simulink model "systeme_sol_2017a_PID_v1"  (R2017a)
settings: Solver=VariableStepAuto  StartTime=0.0  StopTime=50000  RelTol=1e-3
libraries: simulink x2
settings Model: Creator=julien  LastModifiedBy=admin
settings DataIOCC: ReturnWorkspaceOutputs=on
settings SFSimCC: SimUseLocalCustomCode=on
settings RTWCC: RTWUseLocalCustomCode=on

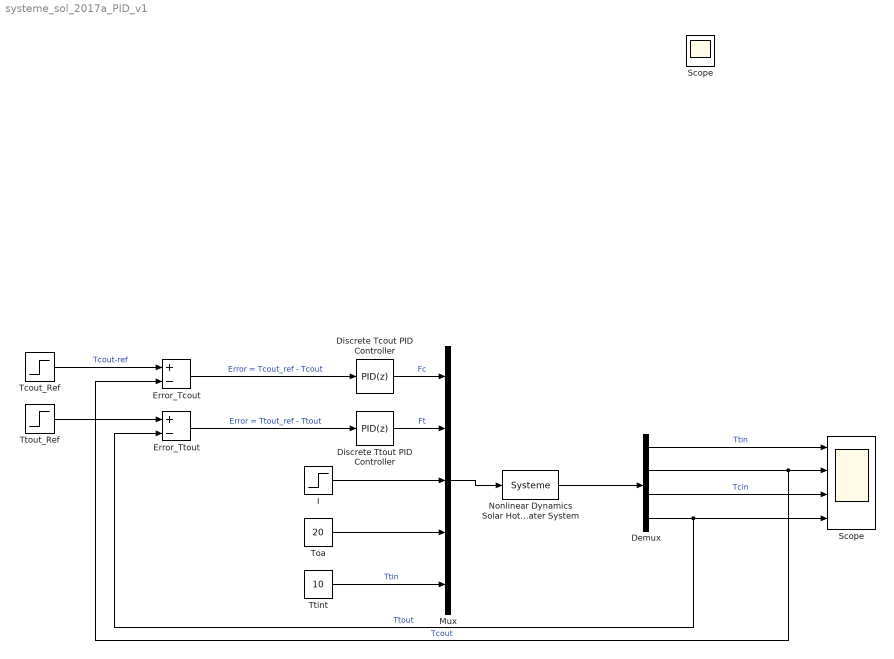
== system systeme_sol_2017a_PID_v1 ==
  Demux : Demux
  Discrete Tcout PID Controller : simulink/Continuous/PID Controller  Controller=PID  TimeDomain=Discrete-time  SampleTime=-1  IntegratorMethod=Forward Euler  FilterMethod=Forward Euler  Form=Ideal  UseFilter=on  ControllerParametersSource=internal  P=-0.0001  I=0  D=0  N=100  InitialConditionSource=internal  InitialConditionForIntegrator=0  InitialConditionForFilter=0  ExternalReset=none  LimitOutput=on  UpperSaturationLimit=2.5e-5  LowerSaturationLimit=0  LinearizeAsGain=off  AntiWindupMode=none  Kb=1  TrackingMode=off  Kt=1  PParamMin=[]  PParamMax=[]  IParamMin=[]  IParamMax=[]  DParamMin=[]  DParamMax=[]  NParamMin=[]  NParamMax=[]  KbParamMin=[]  KbParamMax=[]  KtParamMin=[]  KtParamMax=[]  POutMin=[]  POutMax=[]  IOutMin=[]  IOutMax=[]  DOutMin=[]  DOutMax=[]  NOutMin=[]  NOutMax=[]  KbOutMin=[]  KbOutMax=[]  KtOutMin=[]  KtOutMax=[]  IntegratorOutMin=[]  IntegratorOutMax=[]  FilterOutMin=[]  FilterOutMax=[]  SumOutMin=[]  SumOutMax=[]  SumI1OutMin=[]  SumI1OutMax=[]  SumI2OutMin=[]  SumI2OutMax=[]  SumI3OutMin=[]  SumI3OutMax=[]  SumDOutMin=[]  SumDOutMax=[]  SaturationOutMin=[]  SaturationOutMax=[]  IntegratorContinuousStateAttributes=''  IntegratorStateMustResolveToSignalObject=off  IntegratorRTWStateStorageClass=Auto  FilterContinuousStateAttributes=''  FilterStateMustResolveToSignalObject=off  FilterRTWStateStorageClass=Auto  DifferentiatorICPrevScaledInput=0  DifferentiatorOutMin=[]  DifferentiatorOutMax=[]  InitialConditionSetting=State (most efficient)
  Discrete Ttout PID Controller : simulink/Continuous/PID Controller  Controller=PID  TimeDomain=Discrete-time  SampleTime=-1  IntegratorMethod=Forward Euler  FilterMethod=Forward Euler  Form=Parallel  UseFilter=on  ControllerParametersSource=internal  P=-0.00004  I=0  D=0  N=100  InitialConditionSource=internal  InitialConditionForIntegrator=0  InitialConditionForFilter=0  ExternalReset=none  LimitOutput=on  UpperSaturationLimit=2.5e-5  LowerSaturationLimit=0  LinearizeAsGain=off  AntiWindupMode=none  Kb=1  TrackingMode=off  Kt=1  PParamMin=[]  PParamMax=[]  IParamMin=[]  IParamMax=[]  DParamMin=[]  DParamMax=[]  NParamMin=[]  NParamMax=[]  KbParamMin=[]  KbParamMax=[]  KtParamMin=[]  KtParamMax=[]  POutMin=[]  POutMax=[]  IOutMin=[]  IOutMax=[]  DOutMin=[]  DOutMax=[]  NOutMin=[]  NOutMax=[]  KbOutMin=[]  KbOutMax=[]  KtOutMin=[]  KtOutMax=[]  IntegratorOutMin=[]  IntegratorOutMax=[]  FilterOutMin=[]  FilterOutMax=[]  SumOutMin=[]  SumOutMax=[]  SumI1OutMin=[]  SumI1OutMax=[]  SumI2OutMin=[]  SumI2OutMax=[]  SumI3OutMin=[]  SumI3OutMax=[]  SumDOutMin=[]  SumDOutMax=[]  SaturationOutMin=[]  SaturationOutMax=[]  IntegratorContinuousStateAttributes=''  IntegratorStateMustResolveToSignalObject=off  IntegratorRTWStateStorageClass=Auto  FilterContinuousStateAttributes=''  FilterStateMustResolveToSignalObject=off  FilterRTWStateStorageClass=Auto  DifferentiatorICPrevScaledInput=0  DifferentiatorOutMin=[]  DifferentiatorOutMax=[]  InitialConditionSetting=State (most efficient)
  "Error_Tcout " : Sum  Inputs=+-
  Error_Ttout : Sum  Inputs=+-
  I : Step  Time=50000  Before=1000  After=1000  SampleTime=0
  Mux : Mux  Inputs=5
  Nonlinear Dynamics Solar Hot Water System : S-Function  FunctionName=Systeme  Parameters=60,27.5,47.5  SFunctionDeploymentMode=off  EnableBusSupport=off
  "Scope " : Scope  NumInputPorts=4
  "Tcout_Ref " : Step  Time=20000  Before=60  After=63  SampleTime=0
  Toa : Constant  Value=20
  Ttint : Constant  Value=10
  "Ttout_Ref " : Step  Time=20000  Before=52.5  After=47.5  SampleTime=0
  Scope : Scope
  wires:
  Error_Ttout/1 -> Discrete Ttout PID Controller/1  "Error = Ttout_ref - Ttout"
  I/1 -> Mux/3
  Toa/1 -> Mux/4
  Ttint/1 -> Mux/5  "Ttin"
  Mux/1 -> Nonlinear Dynamics Solar Hot Water System/1
  Nonlinear Dynamics Solar Hot Water System/1 -> Demux/1
  Demux/4 -> Error_Ttout/2, "Scope "/4  "Ttout"
  Demux/3 -> "Scope "/3  "Tcin"
  Demux/2 -> "Error_Tcout "/2, "Scope "/2  "Tcout"
  Demux/1 -> "Scope "/1  "Ttin"
  "Error_Tcout "/1 -> Discrete Tcout PID Controller/1  "Error = Tcout_ref - Tcout"
  "Tcout_Ref "/1 -> "Error_Tcout "/1  "Tcout-ref"
  "Ttout_Ref "/1 -> Error_Ttout/1
  Discrete Ttout PID Controller/1 -> Mux/2  "Ft"
  Discrete Tcout PID Controller/1 -> Mux/1  "Fc"
